simulink model "ce1"  (R2018b)
settings: Solver=VariableStepAuto  StartTime=0.0  StopTime=Tend  FixedStep=Te  RelTol=1e-3
values from neighbouring files (symbols this model uses):
  saturation_limit = 0.5    [ce1_11.m]    (also in ce1_init.m; init.m)
  Te = 0.5    [ce1_11.m]    (also in ce1_3.m; ce1_5.m; ce1_init.m; init.m)
settings Model: Creator=arne  LastModifiedBy=arne

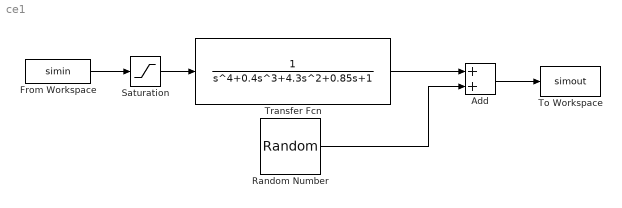
== system ce1 ==
  Add : Sum
  From Workspace : FromWorkspace  VariableName=simin  SampleTime=Te
  Random Number : RandomNumber  Variance=0.01  SampleTime=Te
  Saturation : Saturate  UpperLimit=saturation_limit  LowerLimit=-saturation_limit
  To Workspace : ToWorkspace  VariableName=simout  SaveFormat=Timeseries  SampleTime=Te
  Transfer Fcn : TransferFcn  Denominator=[1 0.4 4.3 0.85 1]
  wires:
  Saturation/1 -> Transfer Fcn/1
  Transfer Fcn/1 -> Add/1
  From Workspace/1 -> Saturation/1
  Add/1 -> To Workspace/1
  Random Number/1 -> Add/2
